simulink model "linear_1_dof_quasi_static_discrete"  (Simulink 7.7)
settings: Solver=ode45  StartTime=0.0  StopTime=50  RelTol=1e-6
values from neighbouring files (symbols this model uses):
  f_thresh = 1000    [matlab_start.m]
  gamma = 7    [matlab_start.m]
  k1 = 10    [matlab_start.m]
  k2 = 10    [matlab_start.m]
  k_a = 10    [matlab_start.m]
  kd = 0    [matlab_start.m]
  ki = 30.025    [matlab_start.m]
  kp = 0.15013    [matlab_start.m]
  t_s = 0.01    [matlab_start.m]
libraries: simulink x3, mpclib x2, commnoisgen2 x1
settings Model: Creator=mkillpack  LastModifiedBy=mkillpack
settings SolverCC: MaxConsecutiveMinStep=3  ZeroCrossAlgorithm=Adaptive  AlgebraicLoopSolver=LineSearch
settings OptimizationCC: SimCompilerOptimization=On

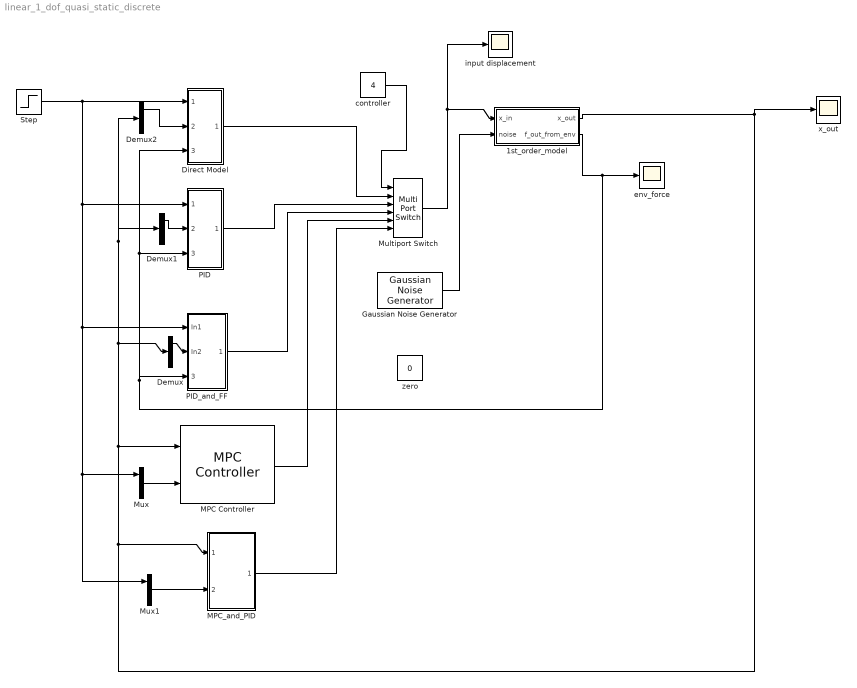
== system linear_1_dof_quasi_static_discrete ==
  1st_order_model : Subsystem
  Demux : Demux  Outputs=2
  Demux1 : Demux  Outputs=2
  Demux2 : Demux  Outputs=2
  Direct Model : Subsystem
  Gaussian Noise Generator : commnoisgen2/Gaussian Noise Generator  SystemSampleTime=-1  m=10  d=2  s=0  Ts=t_s  frameBased=off  sampPerFrame=1  orient=off  outDataType=double
  MPC Controller : mpclib/MPC Controller  SystemSampleTime=-1  mpcobj=MPC1  n_mv=0  x0=[]  ref_from_ws=off  ref_signal_name=[]  ref_preview=on  md_from_ws=off  md_signal_name=[]  md_preview=on  from_project=off  md_inport=off  mv_inport=off  lims_inport=off  switch_inport=off  enable_value=0  project_file=MPCtask.mat  is_multiple=0  cost_outport=off  return_sequence=off
  MPC_and_PID : Subsystem
  Multiport Switch : MultiPortSwitch  Inputs=5  zeroidx=off  SampleTime=t_s
  Mux : Mux  Inputs=2
  Mux1 : Mux  Inputs=2
  PID : Subsystem
  PID_and_FF : Subsystem
  Step : Step  SampleTime=t_s
  controller : Constant  Value=4
  env_force : Scope
      settings: YMin=0  YMax=11  SaveName=ScopeData2
  input displacement : Scope
  x_out : Scope
      settings: YMin=0  YMax=2  SaveName=ScopeData3
  zero : Constant  Value=0
  wires:
  1st_order_model/1(x_out) -> x_out/1, MPC_and_PID/1(x_out), MPC Controller/1, Demux/1, Demux1/1, Demux2/1
  1st_order_model/2(f_out_from_env) -> env_force/1, PID_and_FF/3(f_ext), PID/3(f_ext), Direct Model/3(f_ext)
  Step/1 -> Direct Model/1(In1), PID_and_FF/1(In1), Mux/1, Mux1/1, PID/1(In1)
  Direct Model/1(Out1) -> Multiport Switch/2
  Multiport Switch/1 -> 1st_order_model/1(x_in), input displacement/1
  controller/1 -> Multiport Switch/1
  PID/1(Out1) -> Multiport Switch/3
  PID_and_FF/1(Out1) -> Multiport Switch/4
  Gaussian Noise Generator/1 -> 1st_order_model/2(noise)
  MPC Controller/1 -> Multiport Switch/5
  MPC_and_PID/1(Out1) -> Multiport Switch/6
  Demux/1 -> PID_and_FF/2(In2)
  Demux1/1 -> PID/2(In2)
  Demux2/1 -> Direct Model/2(In2)
  Mux/1 -> MPC Controller/2
  Mux1/1 -> MPC_and_PID/2(x_ref)

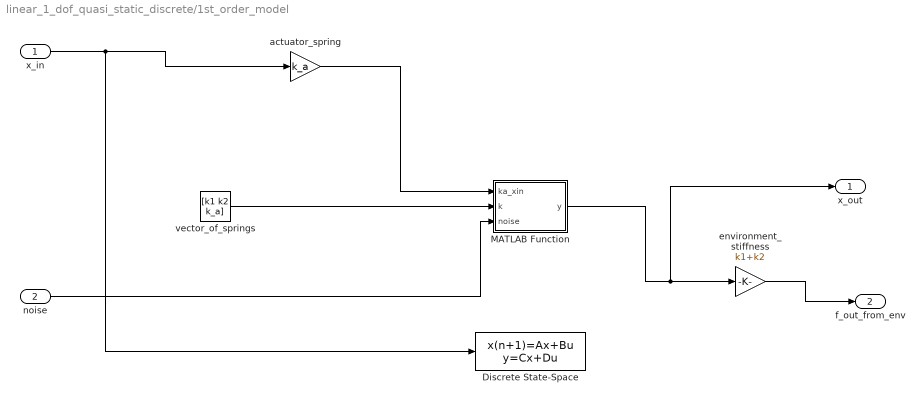
== system linear_1_dof_quasi_static_discrete/1st_order_model ==
  x_in : Inport
  noise : Inport  Port=2
  Discrete State-Space : DiscreteStateSpace  A=0  B=k_a/(k1+k2+k_a)  D=0  SampleTime=.01
  MATLAB Function : Stateflow chart  TreatAsAtomicUnit=on
  actuator_spring : Gain  Gain=k_a
  environment_stiffness : Gain  Gain=k1+k2
  vector_of_springs : Constant  Value=[k1 k2 k_a]
  x_out : Outport
  f_out_from_env : Outport  Port=2
  wires:
  vector_of_springs/1 -> MATLAB Function/2(k)
  noise/1 -> MATLAB Function/3(noise)
  environment_stiffness/1 -> f_out_from_env/1
  x_in/1 -> actuator_spring/1, Discrete State-Space/1
  actuator_spring/1 -> MATLAB Function/1(ka_xin)
  MATLAB Function/1(y) -> environment_stiffness/1, x_out/1

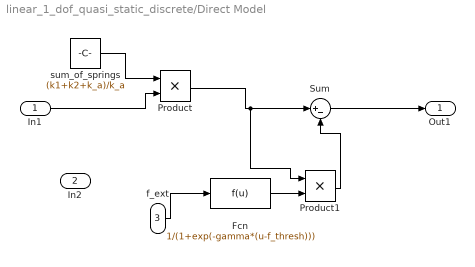
== system linear_1_dof_quasi_static_discrete/Direct Model ==
  In1 : Inport
  In2 : Inport  Port=2
  f_ext : Inport  Port=3
  Fcn : Fcn  Expr=1/(1+exp(-gamma*(u-f_thresh)))
  Product : Product  SampleTime=t_s  RndMeth=Zero
  Product1 : Product  RndMeth=Zero
  Sum : Sum  Inputs=|+-
  sum_of_springs : Constant  Value=(k1+k2+k_a)/k_a
  Out1 : Outport
  wires:
  In1/1 -> Product/2
  sum_of_springs/1 -> Product/1
  Product/1 -> Product1/1, Sum/1
  Sum/1 -> Out1/1
  f_ext/1 -> Fcn/1
  Fcn/1 -> Product1/2
  Product1/1 -> Sum/2

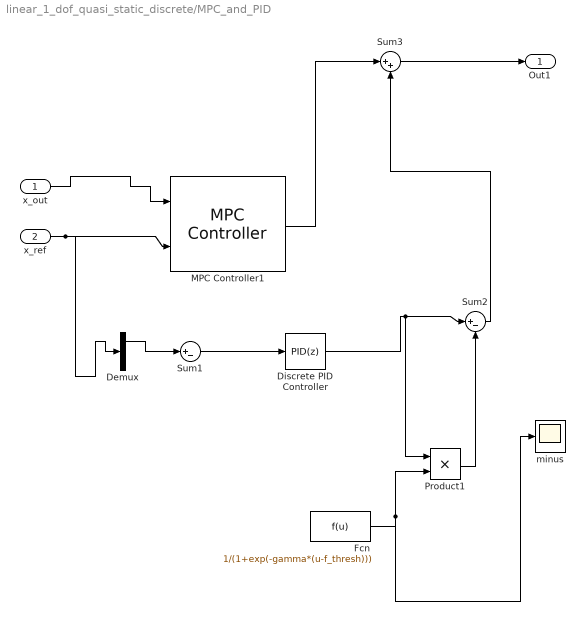
== system linear_1_dof_quasi_static_discrete/MPC_and_PID ==
  x_out : Inport
  x_ref : Inport  Port=2
  Demux : Demux  Outputs=2
  Discrete PID Controller : simulink/Continuous/PID Controller  SystemSampleTime=-1  Controller=PID  TimeDomain=Discrete-time  SampleTime=t_s  IntegratorMethod=Forward Euler  FilterMethod=Forward Euler  Form=Parallel  P=kp  I=ki  D=kd  N=100  InitialConditionSource=internal  InitialConditionForIntegrator=0  InitialConditionForFilter=0  ExternalReset=none  LimitOutput=off  UpperSaturationLimit=inf  LowerSaturationLimit=-inf  LinearizeAsGain=off  AntiWindupMode=none  Kb=1  TrackingMode=off  Kt=1  PParamMin=[]  PParamMax=[]  IParamMin=[]  IParamMax=[]  DParamMin=[]  DParamMax=[]  NParamMin=[]  NParamMax=[]  KbParamMin=[]  KbParamMax=[]  KtParamMin=[]  KtParamMax=[]  POutMin=[]  POutMax=[]  IOutMin=[]  IOutMax=[]  DOutMin=[]  DOutMax=[]  NOutMin=[]  NOutMax=[]  KbOutMin=[]  KbOutMax=[]  KtOutMin=[]  KtOutMax=[]  IntegratorOutMin=[]  IntegratorOutMax=[]  FilterOutMin=[]  FilterOutMax=[]  SumOutMin=[]  SumOutMax=[]  SumI1OutMin=[]  SumI1OutMax=[]  SumI2OutMin=[]  SumI2OutMax=[]  SumI3OutMin=[]  SumI3OutMax=[]  SumDOutMin=[]  SumDOutMax=[]  SaturationOutMin=[]  SaturationOutMax=[]  IntegratorContinuousStateAttributes=''  IntegratorStateMustResolveToSignalObject=off  IntegratorRTWStateStorageClass=Auto  FilterContinuousStateAttributes=''  FilterStateMustResolveToSignalObject=off  FilterRTWStateStorageClass=Auto
  Fcn : Fcn  Expr=1/(1+exp(-gamma*(u-f_thresh)))  SampleTime=t_s
  MPC Controller1 : mpclib/MPC Controller  SystemSampleTime=-1  mpcobj=MPC1  n_mv=0  x0=[]  ref_from_ws=off  ref_signal_name=[]  ref_preview=on  md_from_ws=off  md_signal_name=[]  md_preview=on  from_project=off  md_inport=off  mv_inport=off  lims_inport=off  switch_inport=off  enable_value=0  project_file=MPCtask.mat  is_multiple=0  cost_outport=off  return_sequence=off
  Product1 : Product  RndMeth=Zero
  Sum1 : Sum  Inputs=|+-
  Sum2 : Sum  Inputs=|+-
  Sum3 : Sum  Inputs=|++
  minus : Scope
      settings: YMin=6  YMax=25  SaveName=ScopeData4
  Out1 : Outport
  wires:
  Sum1/1 -> Discrete PID Controller/1
  x_out/1 -> MPC Controller1/1
  x_ref/1 -> MPC Controller1/2, Demux/1
  MPC Controller1/1 -> Sum3/1
  Sum3/1 -> Out1/1
  Fcn/1 -> Product1/2, minus/1
  Product1/1 -> Sum2/2
  Discrete PID Controller/1 -> Sum2/1, Product1/1
  Sum2/1 -> Sum3/2
  Demux/1 -> Sum1/1

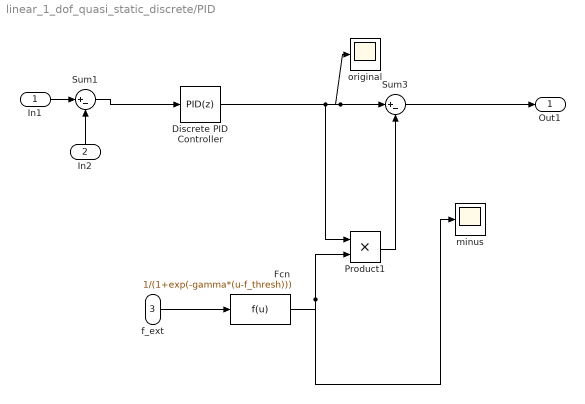
== system linear_1_dof_quasi_static_discrete/PID ==
  In1 : Inport
  In2 : Inport  Port=2
  f_ext : Inport  Port=3
  Discrete PID Controller : simulink/Continuous/PID Controller  SystemSampleTime=-1  Controller=PID  TimeDomain=Discrete-time  SampleTime=t_s  IntegratorMethod=Forward Euler  FilterMethod=Forward Euler  Form=Parallel  P=kp  I=ki  D=kd  N=100  InitialConditionSource=internal  InitialConditionForIntegrator=0  InitialConditionForFilter=0  ExternalReset=none  LimitOutput=off  UpperSaturationLimit=inf  LowerSaturationLimit=-inf  LinearizeAsGain=off  AntiWindupMode=none  Kb=1  TrackingMode=off  Kt=1  PParamMin=[]  PParamMax=[]  IParamMin=[]  IParamMax=[]  DParamMin=[]  DParamMax=[]  NParamMin=[]  NParamMax=[]  KbParamMin=[]  KbParamMax=[]  KtParamMin=[]  KtParamMax=[]  POutMin=[]  POutMax=[]  IOutMin=[]  IOutMax=[]  DOutMin=[]  DOutMax=[]  NOutMin=[]  NOutMax=[]  KbOutMin=[]  KbOutMax=[]  KtOutMin=[]  KtOutMax=[]  IntegratorOutMin=[]  IntegratorOutMax=[]  FilterOutMin=[]  FilterOutMax=[]  SumOutMin=[]  SumOutMax=[]  SumI1OutMin=[]  SumI1OutMax=[]  SumI2OutMin=[]  SumI2OutMax=[]  SumI3OutMin=[]  SumI3OutMax=[]  SumDOutMin=[]  SumDOutMax=[]  SaturationOutMin=[]  SaturationOutMax=[]  IntegratorContinuousStateAttributes=''  IntegratorStateMustResolveToSignalObject=off  IntegratorRTWStateStorageClass=Auto  FilterContinuousStateAttributes=''  FilterStateMustResolveToSignalObject=off  FilterRTWStateStorageClass=Auto
  Fcn : Fcn  Expr=1/(1+exp(-gamma*(u-f_thresh)))  SampleTime=t_s
  Product1 : Product  RndMeth=Zero
  Sum1 : Sum  Inputs=|+-
  Sum3 : Sum  Inputs=|+-
  minus : Scope
      settings: YMin=6  YMax=25
  original : Scope
      settings: SaveName=ScopeData5
  Out1 : Outport
  wires:
  Sum1/1 -> Discrete PID Controller/1
  In2/1 -> Sum1/2
  In1/1 -> Sum1/1
  f_ext/1 -> Fcn/1
  Discrete PID Controller/1 -> Product1/1, Sum3/1, original/1
  Sum3/1 -> Out1/1
  Fcn/1 -> Product1/2, minus/1
  Product1/1 -> Sum3/2

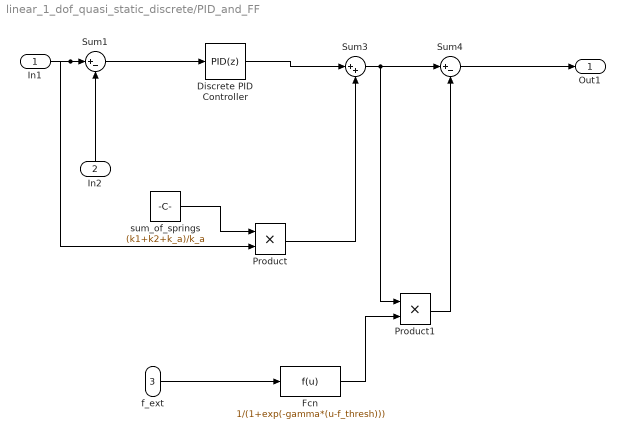
== system linear_1_dof_quasi_static_discrete/PID_and_FF ==
  In1 : Inport
  In2 : Inport  Port=2
  f_ext : Inport  Port=3
  Discrete PID Controller : simulink/Continuous/PID Controller  SystemSampleTime=-1  Controller=PID  TimeDomain=Discrete-time  SampleTime=t_s  IntegratorMethod=Forward Euler  FilterMethod=Forward Euler  Form=Parallel  P=kp  I=ki  D=kd  N=100  InitialConditionSource=internal  InitialConditionForIntegrator=0  InitialConditionForFilter=0  ExternalReset=none  LimitOutput=off  UpperSaturationLimit=inf  LowerSaturationLimit=-inf  LinearizeAsGain=off  AntiWindupMode=none  Kb=1  TrackingMode=off  Kt=1  PParamMin=[]  PParamMax=[]  IParamMin=[]  IParamMax=[]  DParamMin=[]  DParamMax=[]  NParamMin=[]  NParamMax=[]  KbParamMin=[]  KbParamMax=[]  KtParamMin=[]  KtParamMax=[]  POutMin=[]  POutMax=[]  IOutMin=[]  IOutMax=[]  DOutMin=[]  DOutMax=[]  NOutMin=[]  NOutMax=[]  KbOutMin=[]  KbOutMax=[]  KtOutMin=[]  KtOutMax=[]  IntegratorOutMin=[]  IntegratorOutMax=[]  FilterOutMin=[]  FilterOutMax=[]  SumOutMin=[]  SumOutMax=[]  SumI1OutMin=[]  SumI1OutMax=[]  SumI2OutMin=[]  SumI2OutMax=[]  SumI3OutMin=[]  SumI3OutMax=[]  SumDOutMin=[]  SumDOutMax=[]  SaturationOutMin=[]  SaturationOutMax=[]  IntegratorContinuousStateAttributes=''  IntegratorStateMustResolveToSignalObject=off  IntegratorRTWStateStorageClass=Auto  FilterContinuousStateAttributes=''  FilterStateMustResolveToSignalObject=off  FilterRTWStateStorageClass=Auto
  Fcn : Fcn  Expr=1/(1+exp(-gamma*(u-f_thresh)))
  Product : Product  RndMeth=Zero
  Product1 : Product  RndMeth=Zero
  Sum1 : Sum  Inputs=|+-
  Sum3 : Sum  Inputs=|++
  Sum4 : Sum  Inputs=|+-
  sum_of_springs : Constant  Value=(k1+k2+k_a)/k_a
  Out1 : Outport
  wires:
  In2/1 -> Sum1/2
  In1/1 -> Sum1/1, Product/2
  Sum3/1 -> Product1/1, Sum4/1
  sum_of_springs/1 -> Product/1
  Product/1 -> Sum3/2
  f_ext/1 -> Fcn/1
  Fcn/1 -> Product1/2
  Product1/1 -> Sum4/2
  Sum4/1 -> Out1/1
  Sum1/1 -> Discrete PID Controller/1
  Discrete PID Controller/1 -> Sum3/1

== matlab function 1st_order_model/MATLAB Function ==
  data: ka_xin input double; k input double; y output double; noise input double
function y = fcn(ka_xin, k, noise)
%#codegen

y = ka_xin/(k(1)+k(2)+k(3)+noise);
